simulink model "solar_MPPT_bat_charger"  (R2019b)
settings: Solver=VariableStepAuto  StartTime=0.0  StopTime=10.0  RelTol=1e-3
undefined symbols (not defined in the file or in its folder): Acid, Lead, sigbuilder_block
libraries: powerlib x15, powerlib_meascontrol x2, electricdrivelib x1, simulink x1, re_lib x1
settings Model: Creator=root  LastModifiedBy=root

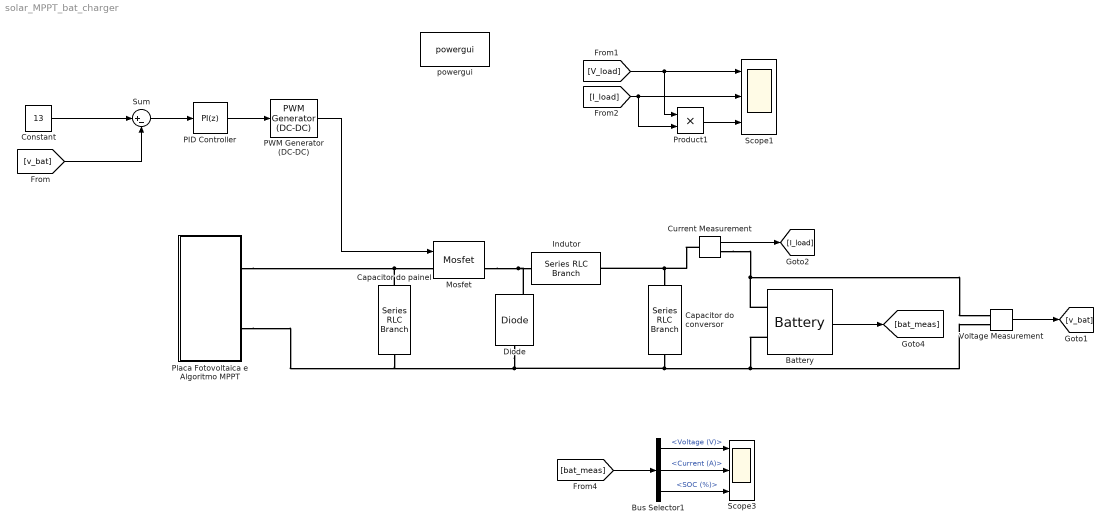
== system solar_MPPT_bat_charger ==
  Battery : electricdrivelib/Extra Sources/Battery  BatType=Lead-Acid  ShowTempParam=off  ThermalPreset=no  ShowAgeParam=off  NomV=12.2  NomQ=240  SOC=40  Batt_Tr=1  PresetModel=on  MaxQ=250  MinV=9.15  FullV=13.2836  Dis_rate=48  R=0.00050833  Normal_OP=74.4667  expZone="[12.4207          0.8]"  current=[6.5 13 32.5]  Units=Time  Tci=20  NomT=20  T2=-30  MaxQ2=4.8  FullV2=7.1  Normal_OP2=5.655  expZone2="[6.58           1]"  Rca=0.6  ti=2000  Dp=0  Neq0=0  Tsim=1e6  Ta1=25  Qeol=5.4*0.9  Reol=0.013333*1.2  Char_age=[2.3478, 3]  Dis_age=[2.3478, 10]  N1=1500  N2=10500  N3=1000  N4=1400  Ta2=45  N5=950
      settings: SourceProductName=Simscape Electrical
  Bus Selector1 : BusSelector  OutputSignals=Voltage (V),Current (A),SOC (%)
  Capacitor do conversor : powerlib/Elements/Series RLC Branch  LConnTagsString=__new0  RConnTagsString=__new0  BranchType=C  Resistance=1e-4  Inductance=1e-3  SetiL0=off  InitialCurrent=0  Capacitance=500e-6  Setx0=off  InitialVoltage=0  Measurements=None
      settings: SourceProductName=Simscape Electrical
  Capacitor do painel : powerlib/Elements/Series RLC Branch  LConnTagsString=__new0  RConnTagsString=__new0  BranchType=C  Resistance=1e-4  Inductance=1e-3  SetiL0=off  InitialCurrent=0  Capacitance=100e-6  Setx0=off  InitialVoltage=0  Measurements=None
      settings: SourceProductName=Simscape Electrical
  Constant : Constant  Value=13
  Current Measurement : powerlib/Measurements/Current Measurement  PhasorSimulation=off  OutputType=Complex  PSBequivalent=0
      settings: SourceProductName=Simscape Electrical
  Diode : powerlib/Power Electronics/Diode  Ron=0.001  Lon=0  Vf=0.8  IC=0  UseSnubber=0  Rs=500  Cs=250e-9  Measurements=on
      settings: SourceProductName=Simscape Electrical
  Indutor : powerlib/Elements/Series RLC Branch  LConnTagsString=__new0  RConnTagsString=__new0  BranchType=L  Resistance=1e-4  Inductance=200e-6  SetiL0=on  InitialCurrent=0  Capacitance=100e-6  Setx0=off  InitialVoltage=0  Measurements=None
      settings: SourceProductName=Simscape Electrical
  Mosfet : powerlib/Power Electronics/Mosfet  Ron=0.1  Lon=0  Rd=0.01  Vfd=0  IC=0  Rs=1e5  Cs=inf  Measurements=on
      settings: SourceProductName=Simscape Electrical
  PID Controller : simulink/Continuous/PID Controller  Controller=PI  Form=Parallel  TimeDomain=Discrete-time  SampleTime=-1  IntegratorMethod=Forward Euler  FilterMethod=Forward Euler  ControllerParametersSource=internal  P=1  I=1  D=0  UseFilter=on  N=100  TunerSelectOption=Transfer Function Based (PID Tuner App)  InitialConditionSource=internal  InitialConditionForIntegrator=0  InitialConditionForFilter=0  DifferentiatorICPrevScaledInput=0  ExternalReset=none  TrackingMode=off  Kt=1  LimitOutput=on  UpperSaturationLimit=1  LowerSaturationLimit=0  LinearizeAsGain=on  AntiWindupMode=none  Kb=1  POutMin=[]  POutMax=[]  IOutMin=[]  IOutMax=[]  DOutMin=[]  DOutMax=[]  NOutMin=[]  NOutMax=[]  SumOutMin=[]  SumOutMax=[]  SaturationOutMin=[]  SaturationOutMax=[]  PParamMin=[]  PParamMax=[]  IParamMin=[]  IParamMax=[]  DParamMin=[]  DParamMax=[]  NParamMin=[]  NParamMax=[]  KbParamMin=[]  KbParamMax=[]  KtParamMin=[]  KtParamMax=[]  KbOutMin=[]  KbOutMax=[]  KtOutMin=[]  KtOutMax=[]  IntegratorOutMin=[]  IntegratorOutMax=[]  FilterOutMin=[]  FilterOutMax=[]  SumI1OutMin=[]  SumI1OutMax=[]  SumI2OutMin=[]  SumI2OutMax=[]  SumI3OutMin=[]  SumI3OutMax=[]  SumI4OutMin=[]  SumI4OutMax=[]  SumDOutMin=[]  SumDOutMax=[]  DifferentiatorOutMin=[]  DifferentiatorOutMax=[]  FilterDiffOutCoefMin=[]  FilterDiffOutCoefMax=[]  ReciprocalOutMin=[]  ReciprocalOutMax=[]  SumDenOutMin=[]  SumDenOutMax=[]  SumNumOutMin=[]  SumNumOutMax=[]  DivideOutMin=[]  DivideOutMax=[]  IntegratorContinuousStateAttributes=''  IntegratorStateMustResolveToSignalObject=off  IntegratorRTWStateStorageClass=Auto  FilterContinuousStateAttributes=''  FilterStateMustResolveToSignalObject=off  FilterRTWStateStorageClass=Auto  ParallelPVariant=InternalParameters  IdealPVariant=Disabled  IVariant=InternalParameters  DVariant=Disabled  IntegratorVariant=Discrete  SatVariant=Enabled  AWVariant=Passthrough  PCopyVariant=Disabled  TRVariant=Disabled  FdbkBlocksVariant=Forward  IdealPFdbkVariant=Disabled  SatFdbkVariant=Disabled  DerivativeFilterVariant=Disabled  NVariant=Disabled  NCopyVariant=Disabled_SignalSpec  FilterICVariant=Disabled  IntegratorICVariant=InternalICs  ExternalResetVariant=Disabled  TRSumVariant=Passthrough  SumFdbkVariant=Disabled  SumVariant=Sum_PI
  PWM Generator (DC-DC) : powerlib_meascontrol/Pulse & Signal Generators/PWM Generator (DC-DC)  Fsw=5000  Ts=0
      settings: SourceProductName=Simscape Electrical
  Placa Fotovoltaica e Algoritmo MPPT : Subsystem
  Product1 : Product
  Scope1 : Scope  NumInputPorts=3
  Scope3 : Scope  NumInputPorts=3
  Sum : Sum  Inputs=|+-
  Voltage Measurement : powerlib/Measurements/Voltage Measurement  PhasorSimulation=off  OutputType=Complex  PSBequivalent=0
      settings: SourceProductName=Simscape Electrical
  powergui : powerlib/powergui  Priority=1  SimulationMode=Discrete  SampleTime=1e-6  frequency=60  Iterations=50  frequencyindice=0  Pbase=100e6  ErrMax=1e-4  UnitsV=kV  UnitsW=MW  buscounter=0  FunctionMessages=off  echomessages=off  EnableUseOfTLC=off  CurrentSourceSwitches=off  DisableSnubberDevices=off  DisableRonSwitches=off  DisableVfSwitches=off  DisplayEquations=off  AutomaticDiscreteSolvers=off  SolverType=Tustin/Backward Euler (TBE)  Interpol=off  ExternalGateDelay=off  methode=off  Ts=100  x0status=blocks  SPID=on  SwTol=0  HookPort=off  NonlinearTolerance=1e-4  nMaxIteration=100  ContinueOnMaxIteration=off  RestoreLinks=warning  ResistiveCurrentMeasurement=off  Frange=[0:2:500]  Ylog=off  Xlog=on  ShowGrid=off  save=off  variable=ZData  structure=0  ZoomFFT=off  StartTime=0.0  cycles=1  DisplayStyle=1  fundamental=60  FreqAxis=off  MaxFrequency=1000  frequencyindicesteady=1  RmsSteady=1  display=off
      settings: SourceProductName=Simscape Electrical
  wires:
  [V_load] -> Product1/1, Scope1/1
  [I_load] -> Scope1/2, Product1/2
  Product1/1 -> Scope1/3
  Voltage Measurement/1 -> [v_bat]
  Current Measurement/1 -> [I_load]
  Battery/1 -> [bat_meas]
  [bat_meas] -> Bus Selector1/1
  Bus Selector1/1 -> Scope3/1  "<Voltage (V)>"
  Bus Selector1/2 -> Scope3/2  "<Current (A)>"
  Bus Selector1/3 -> Scope3/3  "<SOC (%)>"
  Constant/1 -> Sum/1
  [v_bat] -> Sum/2
  Sum/1 -> PID Controller/1
  PID Controller/1 -> PWM Generator (DC-DC)/1
  PWM Generator (DC-DC)/1 -> Mosfet/1
  connections:
  Current Measurement/LConn1 -- Capacitor do conversor/LConn1 -- Indutor/LConn1
  Capacitor do conversor/RConn1 -- Battery/LConn2 -- Voltage Measurement/LConn2 -- Capacitor do painel/RConn1 -- Placa Fotovoltaica e Algoritmo MPPT/RConn2 -- Diode/LConn1
  Capacitor do painel/LConn1 -- Mosfet/LConn1 -- Placa Fotovoltaica e Algoritmo MPPT/RConn1
  Current Measurement/RConn1 -- Battery/LConn1 -- Voltage Measurement/LConn1
  Mosfet/RConn1 -- Diode/RConn1 -- Indutor/RConn1

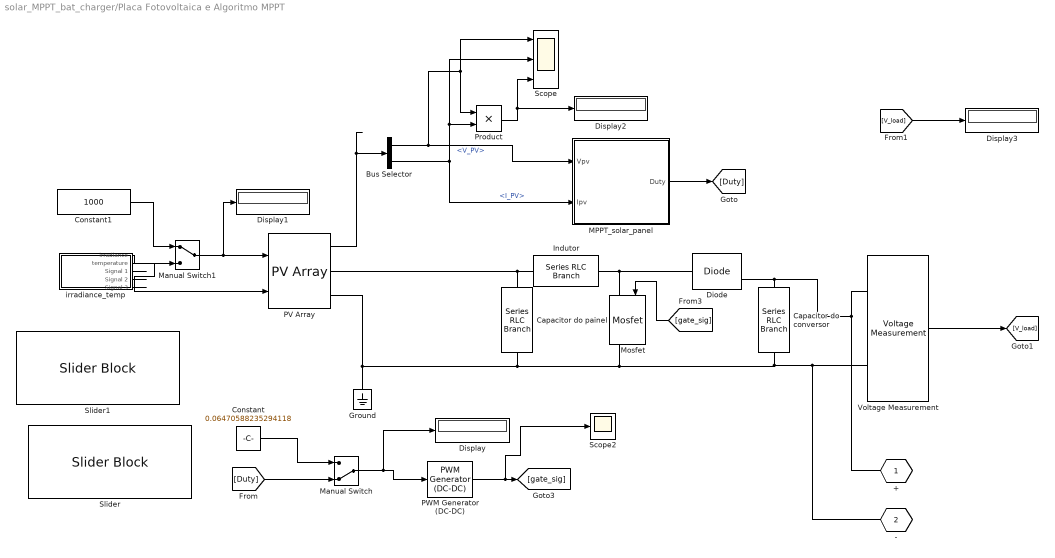
== system solar_MPPT_bat_charger/Placa Fotovoltaica e Algoritmo MPPT ==
  Bus Selector : BusSelector  OutputSignals=V_PV,I_PV
  Capacitor do conversor : powerlib/Elements/Series RLC Branch  LConnTagsString=__new0  RConnTagsString=__new0  BranchType=C  Resistance=1e-4  Inductance=1e-3  SetiL0=off  InitialCurrent=0  Capacitance=500e-6  Setx0=off  InitialVoltage=0  Measurements=None
      settings: SourceProductName=Simscape Electrical
  Capacitor do painel : powerlib/Elements/Series RLC Branch  LConnTagsString=__new0  RConnTagsString=__new0  BranchType=C  Resistance=1e-4  Inductance=1e-3  SetiL0=off  InitialCurrent=0  Capacitance=100e-6  Setx0=off  InitialVoltage=0  Measurements=None
      settings: SourceProductName=Simscape Electrical
  Constant : Constant  Value=0.06470588235294118
  Constant1 : Constant  Value=1000
  Diode : powerlib/Power Electronics/Diode  Ron=0.001  Lon=0  Vf=0.8  IC=0  UseSnubber=0  Rs=500  Cs=250e-9  Measurements=on
      settings: SourceProductName=Simscape Electrical
  Display{,1..3} (4 alike) : Display
  Ground : powerlib/Elements/Ground  LConnTagsString=a
      settings: SourceProductName=Simscape Electrical
  Indutor : powerlib/Elements/Series RLC Branch  LConnTagsString=__new0  RConnTagsString=__new0  BranchType=L  Resistance=1e-4  Inductance=235e-6  SetiL0=off  InitialCurrent=0  Capacitance=100e-6  Setx0=off  InitialVoltage=0  Measurements=None
      settings: SourceProductName=Simscape Electrical
  "MPPT_solar_panel " : MATLAB Function  TreatAsAtomicUnit=on
  Manual Switch : ManualSwitch  CurrentSetting=0
  Manual Switch1 : ManualSwitch
  Mosfet : powerlib/Power Electronics/Mosfet  Ron=0.1  Lon=0  Rd=0.01  Vfd=0  IC=0  Rs=1e5  Cs=inf  Measurements=on
      settings: SourceProductName=Simscape Electrical
  PV Array : re_lib/Solar/PV Array  Npar=1  Nser=1  PlotType=one module @ 25 deg.C & specified irradiances  S_vec="[ 1000  800  600 400 200]"  Temp_C_vec="[ 45 25  ]"  ModuleName=User-defined  PlotWhenSelected=off  Pm=400.488  Ncell=60  Voc=48.70  Isc=10.79  Vm=40.70  Im=9.84  beta_Voc_pc=-0.289  alpha_Isc_pc=0.051  beta_Voc=-0.14074  alpha_Isc=0.0055029  IL=10.8217  I0=2.2788e-11  nI=1.1776  Rsh=79.7466  Rs=0.23394  BAL=on  Tc=1e-6  Tfilter=1e-3
      settings: SourceProductName=Simscape Electrical
  PWM Generator (DC-DC) : powerlib_meascontrol/Pulse & Signal Generators/PWM Generator (DC-DC)  Fsw=30e3  Ts=0
      settings: SourceProductName=Simscape Electrical
  Product : Product
  Scope : Scope  NumInputPorts=3
  Scope2 : Scope
  Slider : SliderBlock  ScaleMax=1
  Slider1 : SliderBlock  ScaleMax=1000
  Voltage Measurement : powerlib/Measurements/Voltage Measurement  PhasorSimulation=off  OutputType=Complex  PSBequivalent=0
      settings: SourceProductName=Simscape Electrical
  irradiance_temp : Subsystem  Tag=STV Subsys  LoadFcn=sigbuilder_block('load');  StartFcn=sigbuilder_block('start');  StopFcn=sigbuilder_block('stop');  ClipboardFcn=sigbuilder_block('clipboard');  mask(Sigbuilder block){tuvar=[0:10]}
      mask help: Simulink:masks:SigbuilderBlock_MD
      mask init:
      | if ~strcmp(get_param(bdroot(gcbh),'SimulationStatus'),'stopped') tuvar = sigbuilder_block('maskInit'); end
      settings: CopyFcn=sigbuilder_block('copy');  DeleteFcn=sigbuilder_block('delete');  ModelCloseFcn=sigbuilder_block('modelClose');  PreSaveFcn=sigbuilder_block('preSave');  PauseFcn=sigbuilder_block('pause');  ContinueFcn=sigbuilder_block('continue');  NameChangeFcn=sigbuilder_block('namechange');  OpenFcn=sigbuilder_block('open',[0 0 1868.11 754.054 ]);  CloseFcn=sigbuilder_block('close');
      mask Display: plot(0, 0, 100, 100,[2, 2, 32, 32, 2], [68, 8, 8, 68, 68],[32, 2], [38, 38], [32, 19, 2],[53, 60, 44], [32, 17, 17, 2],[16, 16, 31, 31]);txt = getActiveGroup(gcbh);text(2, 100, txt,'verticalAlignment', 'top');
  + : PMIOPort  Tag=PMCPort  Side=Right
  - : PMIOPort  Tag=PMCPort  Port=2  Side=Right
  wires:
  Constant/1 -> Manual Switch/1
  [Duty] -> Manual Switch/2
  irradiance_temp/3(Signal 1) -> ?
  PV Array/1 -> Bus Selector/1
  "MPPT_solar_panel "/1(Duty) -> [Duty]
  irradiance_temp/1(irradiance) -> Manual Switch1/2
  Bus Selector/1 -> "MPPT_solar_panel "/1(Vpv), Product/1, Scope/1  "<V_PV>"
  Bus Selector/2 -> "MPPT_solar_panel "/2(Ipv), Scope/2, Product/2  "<I_PV>"
  irradiance_temp/2(temperature) -> PV Array/2
  Manual Switch/1 -> Display/1, PWM Generator (DC-DC)/1
  Manual Switch1/1 -> Display1/1, PV Array/1
  PWM Generator (DC-DC)/1 -> Scope2/1, [gate_sig]
  Constant1/1 -> Manual Switch1/1
  Product/1 -> Display2/1, Scope/3
  irradiance_temp/5(Signal 3) -> ?
  irradiance_temp/4(Signal 2) -> ?
  [gate_sig] -> Mosfet/1
  Voltage Measurement/1 -> [V_load]
  [V_load] -> Display3/1
  connections:
  Indutor/RConn1 -- PV Array/RConn1 -- Capacitor do painel/LConn1
  Diode/RConn1 -- +/RConn1 -- Voltage Measurement/LConn1 -- Capacitor do conversor/LConn1
  Indutor/LConn1 -- Mosfet/LConn1 -- Diode/LConn1
  PV Array/RConn2 -- Capacitor do painel/RConn1 -- -/RConn1 -- Voltage Measurement/LConn2 -- Capacitor do conversor/RConn1 -- Mosfet/RConn1 -- Ground/LConn1

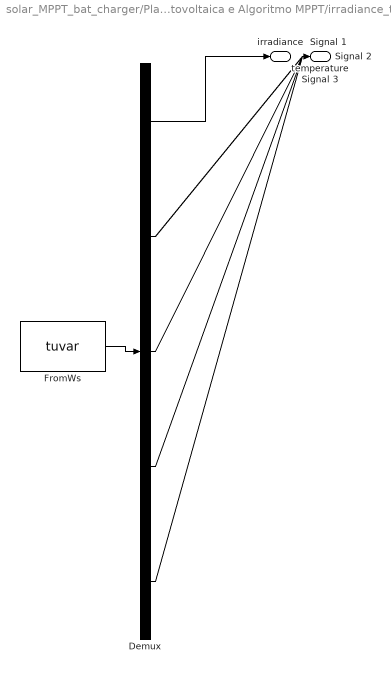
== system solar_MPPT_bat_charger/Placa Fotovoltaica e Algoritmo MPPT/irradiance_temp ==
  Demux : Demux  Tag=STV Demux  Outputs=5
  FromWs : FromWorkspace  Tag=STV FromWs  VariableName=tuvar  SampleTime=0
      SigBuilderData=|
      | common.afterFinalStr = 'Extrapolate'
      | common.sampleTime = 0
      | dataSet.timeRange = [0 10]
      | dataSet.name = 'Group 1'
      | sbobj.Groups.Name = 'Group 1'
      | sbobj.Groups.Signals(1).Name = 'irradiance'
      | sbobj.Groups.Signals(1).XData = [0 1 1.001 2 2.001 3 10]
      | sbobj.Groups.Signals(1).YData = [200 200 400 400 600 1000 1000]
      | sbobj.Groups.Signals(2).Name = 'temperature'
      | sbobj.Groups.Signals(2).XData = [0 5 10]
      | sbobj.Groups.Signals(2).YData = [25 25 25]
      | sbobj.Groups.Signals(3).Name = 'Signal 1'
      | sbobj.Groups.Signals(3).XData = [0 4 4 6 6 10]
      | sbobj.Groups.Signals(3).YData = [0 0 1 1 0 0]
      | sbobj.Groups.Signals(4).Name = 'Signal 2'
      | sbobj.Groups.Signals(4).XData = [0 2 4 6 8 10]
      | sbobj.Groups.Signals(4).YData = [200 400 600 800 900 999]
      | sbobj.Groups.Signals(5).Name = 'Signal 3'
      | sbobj.Groups.Signals(5).XData = [0 1 1 2 2 3 3 4 4 5 5 6 6 7 7 8 8 9 9 10]
      | sbobj.Groups.Signals(5).YData = [0 2 0.12 1.86 0 2 0 2 0 2 0 2 0 2 0 2 0 2 0 2]
  irradiance : Outport  Tag=STV Outport
  temperature : Outport  Tag=STV Outport  Port=2
  Signal 1 : Outport  Tag=STV Outport  Port=3
  Signal 2 : Outport  Tag=STV Outport  Port=4
  Signal 3 : Outport  Tag=STV Outport  Port=5
  wires:
  Demux/1 -> irradiance/1
  FromWs/1 -> Demux/1
  Demux/2 -> temperature/1
  Demux/3 -> Signal 1/1
  Demux/4 -> Signal 2/1
  Demux/5 -> Signal 3/1

== matlab function solar_MPPT_bat_charger/Placa Fotovoltaica e Algoritmo MPPT/MPPT_solar_panel  ==
  data: Vpv input; Duty output; Ipv input
% Codigo para algoritmo MPPT pertubation and observation
% para o painel fotovoltaico.

function Duty = MPPT_solar_panel(Vpv, Ipv)


    %% Declaramos as variaveis do tipo persistent de forma que os valores 
    % fiquem armazenados mesmo com o término da função
    
    persistent Vpv_old Ppv_old Duty_old
    
    % Inicializacao das variaveis
    if isempty(Duty_old)
       Duty_old = 0.5;
       Ppv_old = 0;
       Vpv_old = 0;
    end
    
    Duty_var = 125e-6;           % Delta de variacao a cada iteracao
    
    
    % Calculo do valor de potencia
    
    Ppv = Vpv * Ipv;
    
    %% Inicializacao da comparacao
    
    if ((Ppv - Ppv_old) ~= 0)
       if ((Ppv - Ppv_old) < 0) 
            if ((Vpv - Vpv_old) < 0)
                Duty = Duty_old - Duty_var;
            else 
                Duty = Duty_old + Duty_var;
            end
       else 
           if ((Vpv - Vpv_old) < 0)
                Duty = Duty_old + Duty_var;
           else 
               Duty = Duty_old - Duty_var;
           end
       end
    else 
        
        Duty = Duty_old;
        
    end
    
    if (Duty > 1)
        Duty = 1.0;
    elseif Duty < 0
        Duty = 0.0;
    end 
    
    Ppv_old = Ppv;
    Vpv_old = Vpv;
    Duty_old = Duty;    
end
